simulink model "Drive_ready"  (R2022b)
settings: Solver=FixedStepDiscrete  StartTime=0.0  StopTime=15  FixedStep=0.01  RelTol=1e-3
settings Model: NumberOfSteps=10  PacingRate=1.400000  Creator=12045  LastModifiedBy=12045

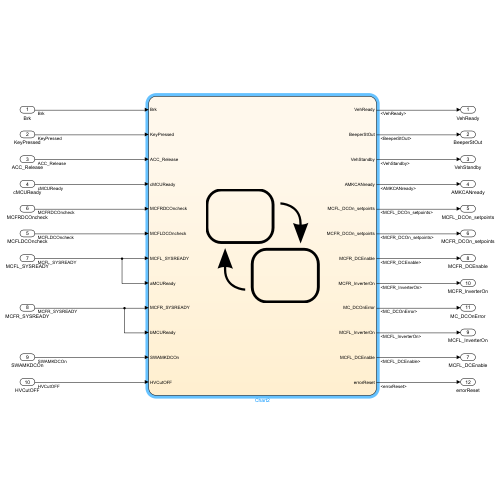
[thumbnail: Simulink's stored preview of the top-level diagram]
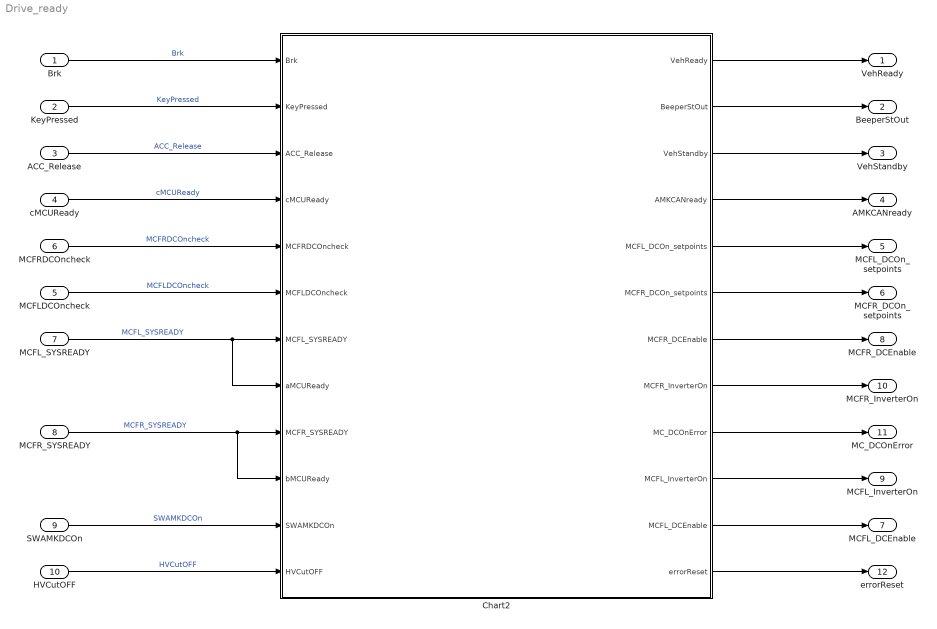
== system Drive_ready ==
  Brk : Inport
  KeyPressed : Inport  Port=2
  ACC_Release : Inport  Port=3
  cMCUReady : Inport  Port=4
  MCFLDCOncheck : Inport  Port=5
  MCFRDCOncheck : Inport  Port=6
  MCFL_SYSREADY : Inport  Port=7
  MCFR_SYSREADY : Inport  Port=8
  SWAMKDCOn : Inport  Port=9
  HVCutOFF : Inport  Port=10
  Chart2 : Stateflow chart  TreatAsAtomicUnit=on
      settings: PortSchema="{\"entries\":[{\"content\":{\"sides\":[{\"content\":{\"connectorIds\":[\"In1\",\"In2\",\"In3\",\"In4\",\"In7\",\"In8\",\"In9\",\"In5\",\"In10\",\"In6\",\"In11\",\"In12\"]},\"type\":\"ConnectorPlacement.EquallySpacedRectSide\",\"uuid\":\"b8fe060c-e9bf-4f00-b6f6-68ec1856d310\"},{\"content\":{\"connectorIds\":[\"Out1\",\"Out2\",\"Out3\",\"Out4\",\"Out5\",\"Out6\",\"Out7\",\"Out8\",\"Out9\",\"Out10\",\"Out11\",\"Out12\"],\"side\":\"RIGHT\"},\"type\":\"ConnectorPlacement.EquallySpacedRectSide\",\"uuid\":\"cc25bea6-df2b-411c-b66d-b7764619fdcc\"},{\"content\":{\"connectorIds\":[],\"side\":\"TOP\"},\"type\":\"ConnectorPlacement.EquallySpacedRectSide\",\"uuid\":\"f8be4ee2-6911-4e67-9b1d-5289fae1a790\"}]},\"type\":\"ConnectorPlacement.EquallySpacedConnector\",\"uuid\":\"1b61a32f-5c0b-4d69-ac60-e1ebfeea406e\"}],\"packageUris\":[\"http://schema.mathworks.com/mf0/Connector/R2020b\"],\"version\":\"1.0\"}"
  VehReady : Outport
  BeeperStOut : Outport  Port=2
  VehStandby : Outport  Port=3
  AMKCANready : Outport  Port=4
  MCFL_DCOn_setpoints : Outport  Port=5
  MCFR_DCOn_setpoints : Outport  Port=6
  MCFL_DCEnable : Outport  Port=7
  MCFR_DCEnable : Outport  Port=8
  MCFL_InverterOn : Outport  Port=9
  MCFR_InverterOn : Outport  Port=10
  MC_DCOnError : Outport  Port=11
  errorReset : Outport  Port=12
  wires:
  Chart2/1(VehReady) -> VehReady/1
  Chart2/2(BeeperStOut) -> BeeperStOut/1
  Chart2/3(VehStandby) -> VehStandby/1
  Chart2/4(AMKCANready) -> AMKCANready/1
  Chart2/5(MCFL_DCOn_setpoints) -> MCFL_DCOn_setpoints/1
  Chart2/6(MCFR_DCOn_setpoints) -> MCFR_DCOn_setpoints/1
  Chart2/11(MCFL_DCEnable) -> MCFL_DCEnable/1
  Chart2/7(MCFR_DCEnable) -> MCFR_DCEnable/1
  Chart2/10(MCFL_InverterOn) -> MCFL_InverterOn/1
  Chart2/8(MCFR_InverterOn) -> MCFR_InverterOn/1
  Chart2/9(MC_DCOnError) -> MC_DCOnError/1
  Brk/1 -> Chart2/1(Brk)  "Brk"
  KeyPressed/1 -> Chart2/2(KeyPressed)  "KeyPressed"
  ACC_Release/1 -> Chart2/3(ACC_Release)  "ACC_Release"
  cMCUReady/1 -> Chart2/4(cMCUReady)  "cMCUReady"
  SWAMKDCOn/1 -> Chart2/11(SWAMKDCOn)  "SWAMKDCOn"
  MCFR_SYSREADY/1 -> Chart2/6(bMCUReady), Chart2/10(MCFR_SYSREADY)  "MCFR_SYSREADY"
  MCFL_SYSREADY/1 -> Chart2/5(aMCUReady), Chart2/9(MCFL_SYSREADY)  "MCFL_SYSREADY"
  MCFRDCOncheck/1 -> Chart2/7(MCFRDCOncheck)  "MCFRDCOncheck"
  MCFLDCOncheck/1 -> Chart2/8(MCFLDCOncheck)  "MCFLDCOncheck"
  HVCutOFF/1 -> Chart2/12(HVCutOFF)  "HVCutOFF"
  Chart2/12(errorReset) -> errorReset/1

== stateflow chart Drive_ready/Chart2 ==
  state VehStat [parallel]
    settings: executionOrder=1
    state WaitForEngine
      en:
      send(AMKCANOFF,AMKCANenable);
      send(AMKDCOFF,AMKDCon);
      send(MCDCEnableOFF,MCDCEnable);
      send(InverterOFF,MC_InverterOn);
    state Standby
    state Trans
    state Guard
    state InitStateBack
    state Ready
    state Init
      en:
      errorReset = 1;
    state MCUReadyFail
    WaitForEngine -> Standby : [aMCUReady&&bMCUReady&&cMCUReady]
    Standby -> Guard [order 2] : [KeyPressed&&Brk&&ACC_Release&&cMCUReady&&aMCUReady&&bMCUReady]
    Trans -> Ready : after(2.5,sec){send(EbeepOFF,BeeperStat)}
    Guard -> Trans [order 1] : after(0.25,sec){send(EbeepON,BeeperStat)}
    Guard -> Standby [order 2] : [~KeyPressed||~Brk||~ACC_Release]
    Standby -> WaitForEngine [order 1] : [~aMCUReady||~bMCUReady||~cMCUReady]
    Guard -> InitStateBack [order 3] : [~cMCUReady||~aMCUReady||~bMCUReady]
    Init -> WaitForEngine : [after(1,sec)]
    MCUReadyFail -> WaitForEngine
    InitStateBack -> WaitForEngine
    Ready -> InitStateBack [order 2] : [~HVCutOFF]
    (default) -> Init
    Ready -> MCUReadyFail [order 1] : [~cMCUReady||~aMCUReady||~bMCUReady]
  state BeeperStat [parallel]
    settings: executionOrder=2
    state OFF
    state ON
    (default) -> BeeperStat.OFF
    BeeperStat.OFF -> BeeperStat.ON : EbeepON
    BeeperStat.ON -> BeeperStat.OFF : EbeepOFF
  state AMKDCon [parallel]
    settings: executionOrder=6
    state OFF
    state ON
    (default) -> AMKDCon.OFF
    AMKDCon.OFF -> AMKDCon.ON : AMKDCON
    AMKDCon.ON -> AMKDCon.OFF : AMKDCOFF
  state MCDCEnable [parallel]
    settings: executionOrder=7
    state OFF
    state ON
    (default) -> MCDCEnable.OFF
    MCDCEnable.OFF -> MCDCEnable.ON : MCDCEnableON
    MCDCEnable.ON -> MCDCEnable.OFF : MCDCEnableOFF
  state AMKDCready [parallel]
    settings: executionOrder=4
    state start
    state AMKCAN
      en:
      send(AMKCANON,AMKCANenable);
    state MC_DCready
    state MCDCOncheck
    state DCOnCheckPass
    state MC_DCOnFail
      en:
      send(AMKDCOFF,AMKDCon);
      send(MCDCEnableOFF,MCDCEnable);
      send(InverterOFF,MC_InverterOn);
    state AMKDCOnFinish
    state SYSRDYCECK
    state MCDCEnableState
      en:
      send(MCDCEnableON,MCDCEnable);
    state MC_InverterOn_State
      en:
      send(InverterON,MC_InverterOn);
    (default) -> start
    AMKCAN -> MC_DCready : [SWAMKDCOn]
    MC_DCready -> MCDCOncheck [order 2] : after(0.1,sec){send(AMKDCON,AMKDCon)}
    MCDCOncheck -> DCOnCheckPass : after(0.1,sec)
    start -> AMKCAN : after(10,sec)
    DCOnCheckPass -> MCDCEnableState [order 1] : after(0.1,sec)[MCFLDCOncheck&&MCFRDCOncheck]
    MC_DCready -> AMKCAN [order 1] : [~SWAMKDCOn]
    DCOnCheckPass -> MC_DCOnFail [order 2] : [~MCFRDCOncheck||~MCFLDCOncheck]
    SYSRDYCECK -> MC_DCOnFail [order 2] : [~MCFL_SYSREADY||~MCFR_SYSREADY]
    SYSRDYCECK -> AMKDCOnFinish [order 1] : [MCFL_SYSREADY&&MCFR_SYSREADY]
    MC_InverterOn_State -> SYSRDYCECK
    MCDCEnableState -> MC_InverterOn_State : after(0.1,sec)
  state Output [parallel]
    du:
    VehReady = in(VehStat.Ready);
    VehStandby = in(VehStat.Standby);
    BeeperStOut = in(BeeperStat.ON);
    AMKCANready = in(AMKCANenable.ON);
    MCFL_DCOn_setpoints = in(AMKDCon.ON);
    MCFR_DCOn_setpoints = in(AMKDCon.ON);
    MCFL_DCEnable = in(MCDCEnable.ON);
    MCFR_DCEnable = in(MCDCEnable.ON);
    MC_DCOnError = in(AMKDCready.MC_DCOnFail);
    MCFL_InverterOn = in(MC_InverterOn.ON);
    MCFR_InverterOn = in(MC_InverterOn.ON);
    settings: executionOrder=3
  state AMKCANenable [parallel]
    settings: executionOrder=5
    state OFF
    state ON
    (default) -> AMKCANenable.OFF
    AMKCANenable.OFF -> AMKCANenable.ON : AMKCANON
    AMKCANenable.ON -> AMKCANenable.OFF : AMKCANOFF
  state MC_InverterOn [parallel]
    settings: executionOrder=8
    state OFF
    state ON
    (default) -> MC_InverterOn.OFF
    MC_InverterOn.OFF -> MC_InverterOn.ON : InverterON
    MC_InverterOn.ON -> MC_InverterOn.OFF : InverterOFF
  data: Brk input boolean size=1; KeyPressed input boolean size=1; VehReady output boolean size=1; BeeperStOut output boolean size=1; VehStandby output boolean; ACC_Release input boolean; cMCUReady input; aMCUReady input; bMCUReady input; AMKCANready output; MCFL_DCOn_setpoints output; MCFRDCOncheck input; MCFLDCOncheck input; MCFR_DCOn_setpoints output; MCFR_DCEnable output; MCFR_InverterOn output; MC_DCOnError output; MCFL_InverterOn output; MCFL_DCEnable output; MCFL_SYSREADY input; MCFR_SYSREADY input; SWAMKDCOn input; HVCutOFF input; errorReset output
  events: EbeepON local FUNCTION_CALL_EVENT; EbeepOFF local FUNCTION_CALL_EVENT; AMKCANOFF local FUNCTION_CALL_EVENT; AMKCANON local FUNCTION_CALL_EVENT; AMKDCON local FUNCTION_CALL_EVENT; AMKDCOFF local FUNCTION_CALL_EVENT; InverterOFF local FUNCTION_CALL_EVENT; InverterON local FUNCTION_CALL_EVENT; MCDCEnableON local FUNCTION_CALL_EVENT; MCDCEnableOFF local FUNCTION_CALL_EVENT
